simulink library "slidercrank_basic_library_v1"  (R2017a)
settings: Solver=VariableStepAuto  StartTime=0.0  StopTime=10.0  RelTol=1e-3
libraries: slidercrank_basic_library_v1 x9
settings Model: Creator=filip  LastModifiedBy=filip

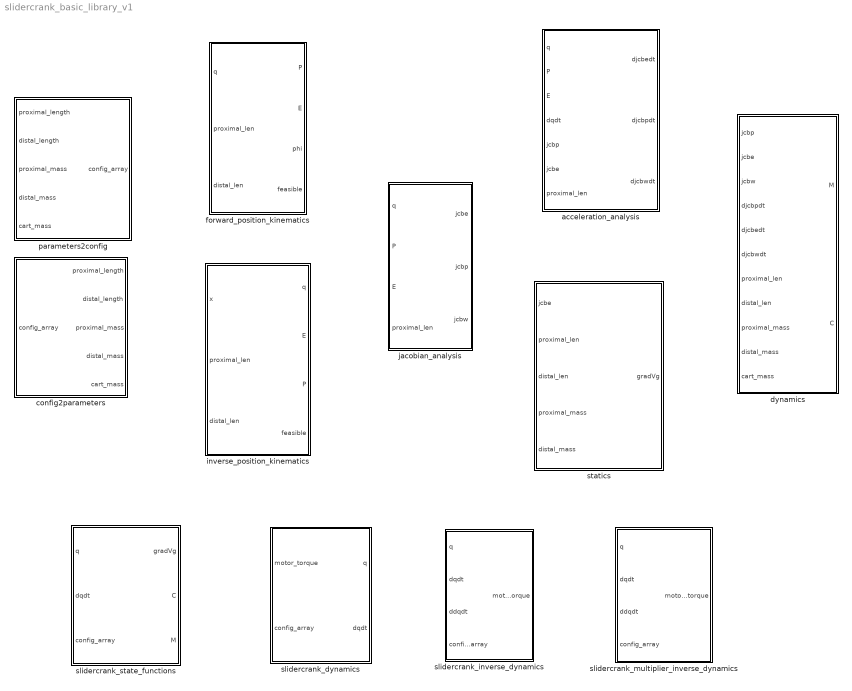
== system slidercrank_basic_library_v1 ==
  acceleration_analysis : Subsystem
  config2parameters : Subsystem
  dynamics : Subsystem
  forward_position_kinematics : Subsystem
  inverse_position_kinematics : Subsystem
  jacobian_analysis : Subsystem
  parameters2config : Subsystem
  slidercrank_dynamics : Subsystem
  slidercrank_inverse_dynamics : Subsystem
  slidercrank_multiplier_inverse_dynamics : Subsystem
  slidercrank_state_functions : Subsystem
  statics : Subsystem

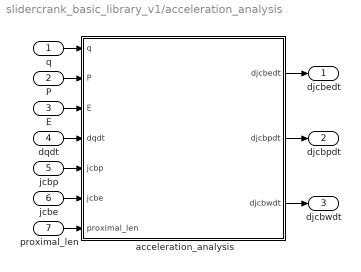
== system slidercrank_basic_library_v1/acceleration_analysis ==
  q : Inport
  P : Inport  Port=2
  E : Inport  Port=3
  dqdt : Inport  Port=4
  jcbp : Inport  Port=5
  jcbe : Inport  Port=6
  proximal_len : Inport  Port=7
  acceleration_analysis : MATLAB Function  TreatAsAtomicUnit=on
  djcbedt : Outport
  djcbpdt : Outport  Port=2
  djcbwdt : Outport  Port=3
  wires:
  acceleration_analysis/1(djcbedt) -> djcbedt/1
  acceleration_analysis/2(djcbpdt) -> djcbpdt/1
  acceleration_analysis/3(djcbwdt) -> djcbwdt/1
  P/1 -> acceleration_analysis/2(P)
  q/1 -> acceleration_analysis/1(q)
  E/1 -> acceleration_analysis/3(E)
  dqdt/1 -> acceleration_analysis/4(dqdt)
  jcbp/1 -> acceleration_analysis/5(jcbp)
  jcbe/1 -> acceleration_analysis/6(jcbe)
  proximal_len/1 -> acceleration_analysis/7(proximal_len)

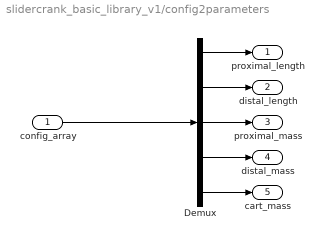
== system slidercrank_basic_library_v1/config2parameters ==
  config_array : Inport
  Demux : Demux  Outputs=5
  proximal_length : Outport
  distal_length : Outport  Port=2
  proximal_mass : Outport  Port=3
  distal_mass : Outport  Port=4
  cart_mass : Outport  Port=5
  wires:
  Demux/1 -> proximal_length/1
  Demux/2 -> distal_length/1
  Demux/3 -> proximal_mass/1
  Demux/4 -> distal_mass/1
  Demux/5 -> cart_mass/1
  config_array/1 -> Demux/1

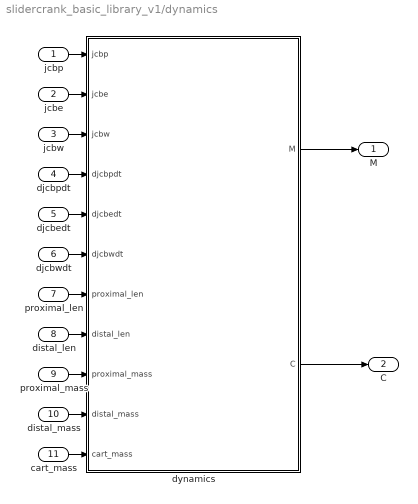
== system slidercrank_basic_library_v1/dynamics ==
  jcbp : Inport
  jcbe : Inport  Port=2
  jcbw : Inport  Port=3
  djcbpdt : Inport  Port=4
  djcbedt : Inport  Port=5
  djcbwdt : Inport  Port=6
  proximal_len : Inport  Port=7
  distal_len : Inport  Port=8
  proximal_mass : Inport  Port=9
  distal_mass : Inport  Port=10
  cart_mass : Inport  Port=11
  dynamics : MATLAB Function  TreatAsAtomicUnit=on
  M : Outport
  C : Outport  Port=2
  wires:
  dynamics/1(M) -> M/1
  dynamics/2(C) -> C/1
  jcbp/1 -> dynamics/1(jcbp)
  jcbe/1 -> dynamics/2(jcbe)
  jcbw/1 -> dynamics/3(jcbw)
  djcbpdt/1 -> dynamics/4(djcbpdt)
  djcbedt/1 -> dynamics/5(djcbedt)
  djcbwdt/1 -> dynamics/6(djcbwdt)
  proximal_len/1 -> dynamics/7(proximal_len)
  distal_len/1 -> dynamics/8(distal_len)
  proximal_mass/1 -> dynamics/9(proximal_mass)
  distal_mass/1 -> dynamics/10(distal_mass)
  cart_mass/1 -> dynamics/11(cart_mass)

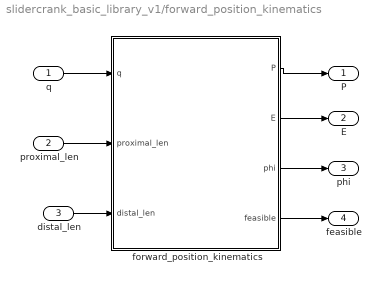
== system slidercrank_basic_library_v1/forward_position_kinematics ==
  q : Inport
  proximal_len : Inport  Port=2
  distal_len : Inport  Port=3
  forward_position_kinematics : MATLAB Function  TreatAsAtomicUnit=on
  P : Outport
  E : Outport  Port=2
  phi : Outport  Port=3
  feasible : Outport  Port=4
  wires:
  q/1 -> forward_position_kinematics/1(q)
  proximal_len/1 -> forward_position_kinematics/2(proximal_len)
  distal_len/1 -> forward_position_kinematics/3(distal_len)
  forward_position_kinematics/1(P) -> P/1
  forward_position_kinematics/2(E) -> E/1
  forward_position_kinematics/4(feasible) -> feasible/1
  forward_position_kinematics/3(phi) -> phi/1

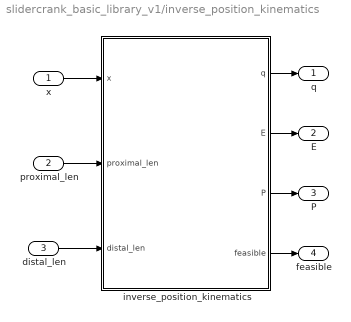
== system slidercrank_basic_library_v1/inverse_position_kinematics ==
  x : Inport
  proximal_len : Inport  Port=2
  distal_len : Inport  Port=3
  inverse_position_kinematics : MATLAB Function  TreatAsAtomicUnit=on
  q : Outport
  E : Outport  Port=2
  P : Outport  Port=3
  feasible : Outport  Port=4
  wires:
  inverse_position_kinematics/1(q) -> q/1
  inverse_position_kinematics/2(E) -> E/1
  inverse_position_kinematics/3(P) -> P/1
  inverse_position_kinematics/4(feasible) -> feasible/1
  x/1 -> inverse_position_kinematics/1(x)
  proximal_len/1 -> inverse_position_kinematics/2(proximal_len)
  distal_len/1 -> inverse_position_kinematics/3(distal_len)

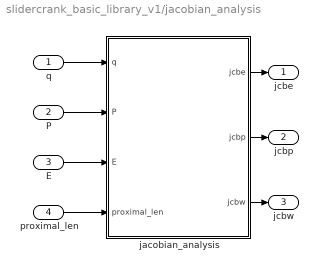
== system slidercrank_basic_library_v1/jacobian_analysis ==
  q : Inport
  P : Inport  Port=2
  E : Inport  Port=3
  proximal_len : Inport  Port=4
  jacobian_analysis : MATLAB Function  TreatAsAtomicUnit=on
  jcbe : Outport
  jcbp : Outport  Port=2
  jcbw : Outport  Port=3
  wires:
  jacobian_analysis/1(jcbe) -> jcbe/1
  jacobian_analysis/2(jcbp) -> jcbp/1
  jacobian_analysis/3(jcbw) -> jcbw/1
  P/1 -> jacobian_analysis/2(P)
  q/1 -> jacobian_analysis/1(q)
  E/1 -> jacobian_analysis/3(E)
  proximal_len/1 -> jacobian_analysis/4(proximal_len)

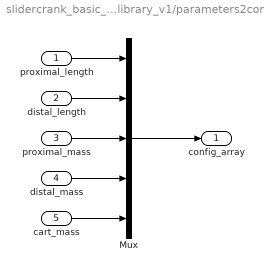
== system slidercrank_basic_library_v1/parameters2config ==
  proximal_length : Inport
  distal_length : Inport  Port=2
  proximal_mass : Inport  Port=3
  distal_mass : Inport  Port=4
  cart_mass : Inport  Port=5
  Mux : Mux  Inputs=5
  config_array : Outport
  wires:
  cart_mass/1 -> Mux/5
  distal_mass/1 -> Mux/4
  proximal_mass/1 -> Mux/3
  distal_length/1 -> Mux/2
  proximal_length/1 -> Mux/1
  Mux/1 -> config_array/1

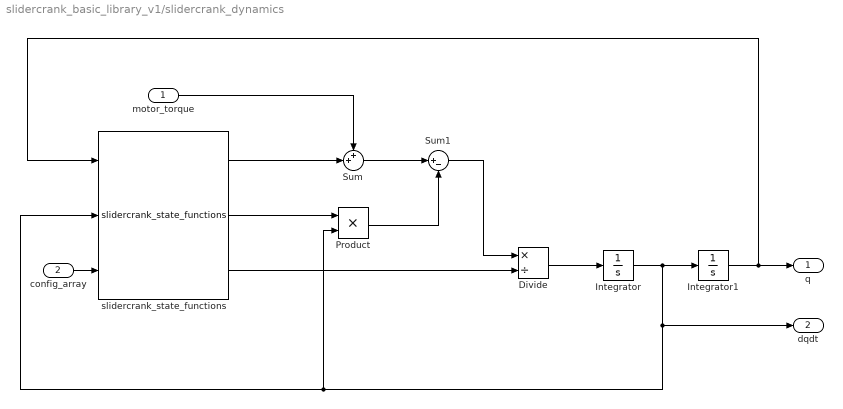
== system slidercrank_basic_library_v1/slidercrank_dynamics ==
  motor_torque : Inport
  config_array : Inport  Port=2
  Divide : Product  Inputs=*/
  Integrator : Integrator
  Integrator1 : Integrator
  Product : Product
  Sum : Sum  Inputs=++|
  Sum1 : Sum  Inputs=|+-
  slidercrank_state_functions : slidercrank_basic_library_v1/slidercrank_state_functions
  q : Outport
  dqdt : Outport  Port=2
  wires:
  slidercrank_state_functions/3 -> Divide/2
  motor_torque/1 -> Sum/1
  slidercrank_state_functions/1 -> Sum/2
  Sum/1 -> Sum1/1
  Product/1 -> Sum1/2
  Sum1/1 -> Divide/1
  Divide/1 -> Integrator/1
  Integrator/1 -> slidercrank_state_functions/2, Product/2, dqdt/1, Integrator1/1
  Integrator1/1 -> slidercrank_state_functions/1, q/1
  slidercrank_state_functions/2 -> Product/1
  config_array/1 -> slidercrank_state_functions/3

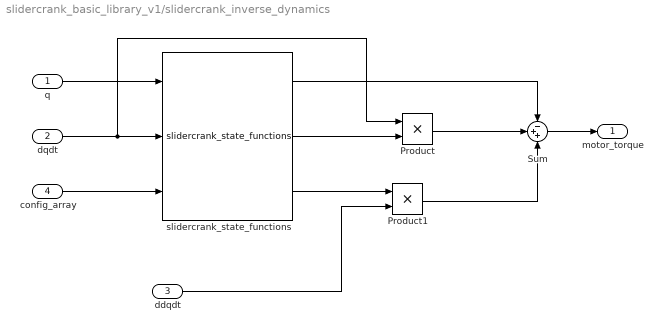
== system slidercrank_basic_library_v1/slidercrank_inverse_dynamics ==
  q : Inport
  dqdt : Inport  Port=2
  ddqdt : Inport  Port=3
  config_array : Inport  Port=4
  Product : Product
  Product1 : Product
  Sum : Sum  Inputs=-++
  slidercrank_state_functions : slidercrank_basic_library_v1/slidercrank_state_functions
  motor_torque : Outport
  wires:
  q/1 -> slidercrank_state_functions/1
  dqdt/1 -> Product/1, slidercrank_state_functions/2
  config_array/1 -> slidercrank_state_functions/3
  slidercrank_state_functions/2 -> Product/2
  slidercrank_state_functions/3 -> Product1/1
  ddqdt/1 -> Product1/2
  Sum/1 -> motor_torque/1
  slidercrank_state_functions/1 -> Sum/1
  Product/1 -> Sum/2
  Product1/1 -> Sum/3

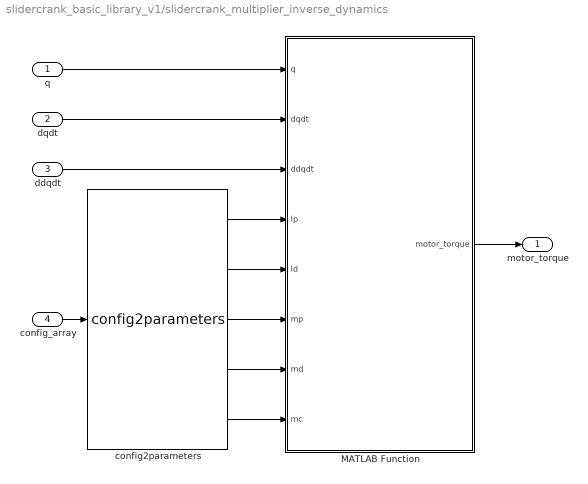
== system slidercrank_basic_library_v1/slidercrank_multiplier_inverse_dynamics ==
  q : Inport
  dqdt : Inport  Port=2
  ddqdt : Inport  Port=3
  config_array : Inport  Port=4
  MATLAB Function : MATLAB Function  TreatAsAtomicUnit=on
  config2parameters : slidercrank_basic_library_v1/config2parameters
  motor_torque : Outport
  wires:
  q/1 -> MATLAB Function/1(q)
  dqdt/1 -> MATLAB Function/2(dqdt)
  ddqdt/1 -> MATLAB Function/3(ddqdt)
  MATLAB Function/1(motor_torque) -> motor_torque/1
  config2parameters/1 -> MATLAB Function/4(lp)
  config2parameters/2 -> MATLAB Function/5(ld)
  config2parameters/3 -> MATLAB Function/6(mp)
  config2parameters/4 -> MATLAB Function/7(md)
  config2parameters/5 -> MATLAB Function/8(mc)
  config_array/1 -> config2parameters/1

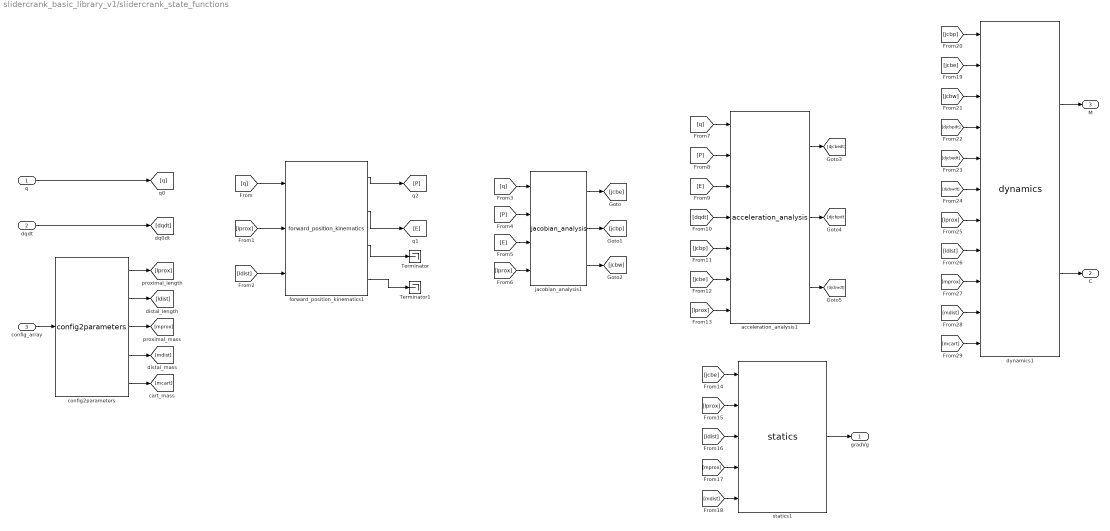
== system slidercrank_basic_library_v1/slidercrank_state_functions ==
  q : Inport
  dqdt : Inport  Port=2
  config_array : Inport  Port=3
  Terminator : Terminator
  Terminator1 : Terminator
  acceleration_analysis1 : slidercrank_basic_library_v1/acceleration_analysis
  config2parameters : slidercrank_basic_library_v1/config2parameters
  dynamics1 : slidercrank_basic_library_v1/dynamics
  forward_position_kinematics1 : slidercrank_basic_library_v1/forward_position_kinematics
  jacobian_analysis1 : slidercrank_basic_library_v1/jacobian_analysis
  statics1 : slidercrank_basic_library_v1/statics
  gradVg : Outport
  C : Outport  Port=2
  M : Outport  Port=3
  wires:
  config_array/1 -> config2parameters/1
  config2parameters/1 -> [lprox]
  config2parameters/2 -> [ldist]
  config2parameters/3 -> [mprox]
  config2parameters/4 -> [mdist]
  config2parameters/5 -> [mcart]
  q/1 -> [q]
  dqdt/1 -> [dqdt]
  [q] -> forward_position_kinematics1/1
  [lprox] -> forward_position_kinematics1/2
  [ldist] -> forward_position_kinematics1/3
  forward_position_kinematics1/2 -> [E]
  forward_position_kinematics1/1 -> [P]
  [q] -> jacobian_analysis1/1
  [P] -> jacobian_analysis1/2
  [E] -> jacobian_analysis1/3
  [lprox] -> jacobian_analysis1/4
  jacobian_analysis1/1 -> [jcbe]
  jacobian_analysis1/2 -> [jcbp]
  jacobian_analysis1/3 -> [jcbw]
  [q] -> acceleration_analysis1/1
  [P] -> acceleration_analysis1/2
  [E] -> acceleration_analysis1/3
  [dqdt] -> acceleration_analysis1/4
  [jcbp] -> acceleration_analysis1/5
  [jcbe] -> acceleration_analysis1/6
  [lprox] -> acceleration_analysis1/7
  acceleration_analysis1/1 -> [djcbedt]
  acceleration_analysis1/2 -> [djcbpdt]
  acceleration_analysis1/3 -> [djcbwdt]
  [jcbe] -> statics1/1
  [lprox] -> statics1/2
  [ldist] -> statics1/3
  [mprox] -> statics1/4
  [mdist] -> statics1/5
  statics1/1 -> gradVg/1
  [jcbe] -> dynamics1/2
  [jcbp] -> dynamics1/1
  [jcbw] -> dynamics1/3
  [djcbpdt] -> dynamics1/4
  [djcbedt] -> dynamics1/5
  [djcbwdt] -> dynamics1/6
  [lprox] -> dynamics1/7
  [ldist] -> dynamics1/8
  [mprox] -> dynamics1/9
  [mdist] -> dynamics1/10
  [mcart] -> dynamics1/11
  dynamics1/2 -> C/1
  dynamics1/1 -> M/1
  forward_position_kinematics1/3 -> Terminator/1
  forward_position_kinematics1/4 -> Terminator1/1

== system slidercrank_basic_library_v1/statics ==
  jcbe : Inport
  proximal_len : Inport  Port=2
  distal_len : Inport  Port=3
  proximal_mass : Inport  Port=4
  distal_mass : Inport  Port=5
  statics : MATLAB Function  TreatAsAtomicUnit=on
  gradVg : Outport
  wires:
  statics/1(grad_Vg) -> gradVg/1
  jcbe/1 -> statics/1(jcbe)
  proximal_len/1 -> statics/2(proximal_len)
  distal_len/1 -> statics/3(distal_len)
  proximal_mass/1 -> statics/4(proximal_mass)
  distal_mass/1 -> statics/5(distal_mass)

== matlab function slidercrank_basic_library_v1/inverse_position_kinematics/inverse_position_kinematics ==
  data: x input; q output; proximal_len input; E output; P output; feasible output; distal_len input
function [q,E,P,feasible] = inverse_position_kinematics(x, proximal_len, distal_len)
    q = 0;
    P = zeros(3,1);
    E = zeros(3,1);
    
    P = [x;0;0];
    O = [0;0;0];
    pt = zeros(2,2);
    [pt(:,1), pt(:,2), nfound] = intersect_circles(O, proximal_len, P, distal_len);
    if (nfound == 0)
        P = NaN(3,1);
        E = NaN(3,1);
        q = NaN(1,1);
        feasible  = false;
    else
        y        = pt(2,:);
        [~,imx]  = max(y);
        E = [pt(1,imx); pt(2,imx); 0];
        q = atan2(E(2),E(1));
        feasible  = true;
    end
end

== matlab function slidercrank_basic_library_v1/slidercrank_multiplier_inverse_dynamics/MATLAB Function ==
  data: q input; motor_torque output; dqdt input; ddqdt input; lp input; ld input; mp input; md input; mc input
function motor_torque  = inverse_dynamics(q, dqdt, ddqdt, lp, ld, mp, md, mc)
%
    [P,E,feasible]            = forward_position_kinematics(q, lp, ld);
    [jcbe,jcbp,jcbw]          = jacobian_analysis(q,P,E,lp);
    [djcbedt,djcbpdt,djcbwdt] = acceleration_analysis(q,P,E,dqdt,jcbp,jcbe,lp);
    
    PE = E - P;
    phi = atan2(PE(2), PE(1));

%   NB: xi = [q,xprox,yprox,phi,xdist,ydist,xcart]'
    gconst = 9.81;
    Jp = mp * lp^2 / 12;
    Jd = md * ld^2 / 12;
    m = [Jp, 
         mp,
         mp,
         Jd,
         md,
         md,
         mc];
    M = diag(m);
    %
    grad_Vg = -gconst * [0; 0; mp; 0; 0; md; 0];
    %
    jcbg1    = jcbe * 0.5;
    jcbg2    = jcbe * 0.5 + jcbp * 0.5;
    djcbg1dt = djcbedt * 0.5;
    djcbg2dt = djcbedt * 0.5 + djcbpdt * 0.5;
    ddG1dt   = jcbg1 * ddqdt + djcbg1dt * dqdt;
    ddG2dt   = jcbg2 * ddqdt + djcbg2dt * dqdt;
    ddPdt    = jcbp * ddqdt + djcbpdt * dqdt;
    ddwdt    = jcbw * ddqdt + djcbwdt * dqdt;

    ddxidt = [ddqdt;
              ddG1dt(1:2);
              ddwdt(3);
              ddG2dt(1:2);
              ddPdt(1)];
    %
    %   jacobian of the constraint equations:
    dCnstr = [-0.5 * lp * sin(q), 1, 0, 0.5 * ld * sin(phi), -1, 0, 0;
               0.5 * lp * cos(q), 0, 1,-0.5 * ld * cos(phi),  0,-1, 0;
               0.5 * lp * sin(q), 1, 0, 0, 0, 0, 0;
              -0.5 * lp * cos(q), 0, 1, 0 ,0, 0, 0;
               0, 0, 0,-0.5*ld * sin(phi),-1, 0, 1;
               0, 0, 0,-0.5*ld * cos(phi), 0, 1, 0];
    %   solution of the inverse dynamics:
    A  = [1,0,0,0,0,0,0;
         dCnstr];
    sol = A' \ (M * ddxidt - grad_Vg);
    motor_torque = sol(1);
end

== matlab function slidercrank_basic_library_v1/jacobian_analysis/jacobian_analysis ==
  data: q input; P input; E input; jcbe output; proximal_len input; jcbp output; jcbw output
function [jcbe,jcbp,jcbw] = jacobian_analysis(q,P,E,proximal_len)
    jcbe = zeros(3,1);
    jcbp = zeros(3,1);
    jcbw = zeros(3,1);
    EP            = P - E;
    jcbe  = proximal_len * [-sin(q); cos(q); 0];
    jcbp  = [dot(jcbe, EP) / EP(1); 0; 0];
    jcbw  = [0; 0;  (jcbp(2) - jcbe(2)) / EP(1)];
end

== matlab function slidercrank_basic_library_v1/acceleration_analysis/acceleration_analysis ==
  data: q input; djcbedt output; P input; E input; dqdt input; jcbp input; jcbe input; proximal_len input; djcbpdt output; djcbwdt output
function [djcbedt,djcbpdt,djcbwdt] = acceleration_analysis(q,P,E,dqdt,jcbp,jcbe,proximal_len)
    djcbedt = zeros(3,1);
    djcbpdt = zeros(3,1);
    djcbwdt = zeros(3,1);
    
    EP              = P - E;
    dpdt            = jcbp * dqdt;
    dedt            = jcbe * dqdt;
    dEPdt           = dpdt - dedt;

    djcbedt = proximal_len * [-cos(q); -sin(q); 0] * dqdt;
%   accelerazione del piede di biella:
    %num    = dot(jcbe, EP);
    num    = jcbe(1) * EP(1) + jcbe(2) * EP(2) + jcbe(3) * EP(3);

    den    = EP(1);
    %dnumdt = dot(djcbedt, EP) + dot(jcbe, dEPdt);c
    dnumdt  = djcbedt(1)*EP(1) + djcbedt(2) * EP(2) + djcbedt(3) * EP(3) +...
              jcbe(1) * dEPdt(1) + jcbe(2) * dEPdt(2) + jcbe(3) * dEPdt(3);
    ddendt = dEPdt(1);
    djcbpdt = [(dnumdt * den - num * ddendt) / den^2; 0; 0];

%   accelerazione angolare della biella:
    num    = jcbp(2) - jcbe(2);
    den    = EP(1);
    dnumdt = djcbpdt(2) - djcbedt(2);
    ddendt = dEPdt(1);
    djcbwdt = [0; 0; (dnumdt * den - num * ddendt) / den^2];
end

== matlab function slidercrank_basic_library_v1/statics/statics ==
  data: jcbe input; grad_Vg output; proximal_len input; distal_len input; proximal_mass input; distal_mass input
function grad_Vg  = statics(jcbe,proximal_len, distal_len, proximal_mass, distal_mass)
%   Output: static torque acting on the system:
    grad_Vg = 0;
    gconst = 9.81;
    grad_y_prox   = 0.5 * jcbe(2);
    grad_y_dist   = 0.5 * jcbe(2);
    grad_Vg       =-gconst * (proximal_mass * grad_y_prox + distal_mass * grad_y_dist);
end

== matlab function slidercrank_basic_library_v1/dynamics/dynamics ==
  data: jcbp input; M output; jcbe input; jcbw input; djcbpdt input; djcbedt input; djcbwdt input; proximal_len input; C output; distal_len input; proximal_mass input; distal_mass input; cart_mass input
function [M,C] = dynamics(jcbp,jcbe,jcbw,djcbpdt,djcbedt,djcbwdt,proximal_len,distal_len,proximal_mass,distal_mass,cart_mass)
    proximal_J = proximal_mass * proximal_len^2 / 12;
    distal_J   = distal_mass * distal_len^2 / 12;

    jcbgp = 0.5 * jcbe;
    jcbgd = 0.5 *jcbe + 0.5 * jcbp;

    djcbgpdt = 0.5 * djcbedt;
    djcbgddt = 0.5 *  djcbedt + 0.5 * djcbpdt;

    Mprox = proximal_J + proximal_mass * (jcbgp.' * jcbgp);
    Mdist = distal_J * (jcbw.' * jcbw) + distal_mass * (jcbgd.' * jcbgd);
    Mcart = cart_mass  * (jcbp.' * jcbp);
    
    Cprox = 0;
    Cdist = 0;
    Ccart = 0;
    C     = 0;
    Cprox = (proximal_mass * (jcbgp.' * djcbgpdt));
    Cdist = (distal_mass * (jcbgd.' * djcbgddt) +...
             distal_J * (jcbw.'  * djcbwdt));
    Ccart = (cart_mass * (jcbp.'  * djcbpdt));

    M = Mprox + Mdist + Mcart;
    C = Cprox + Cdist + Ccart;
end

== matlab function slidercrank_basic_library_v1/forward_position_kinematics/forward_position_kinematics ==
  data: q input; P output; proximal_len input; E output; phi output; feasible output; distal_len input
function [P,E,phi,feasible] = forward_position_kinematics(q, proximal_len, distal_len)
    P = zeros(3,1);
    E = zeros(3,1);
    
    E = proximal_len * [cos(q); sin(q); 0];
    a = 1;
    b =-2 * E(1);
    c = E(1)^2 + E(2)^2 - distal_len^2;

    delta = b^2 - 4*a*c;
    if (delta < 0)
        P = NaN(3,1);
        phi = NaN(1,1);
        feasible  = false;
    else
        x1 = (-b  + sqrt(delta)) / (2*a);
        x2 = (-b  - sqrt(delta)) / (2*a);
        P = [x1; 0; 0]; % an assembly is implied.
        PE = E - P;
        phi = atan2(PE(2),PE(1));
        feasible  = true;
    end
end
